simulink model "MPC3DoF_state_est"  (R2024b)
settings: Solver=VariableStepAuto  StartTime=0.0  StopTime=stop_time  RelTol=1e-3
model workspace (MAT data in the model file):
  com_error = 0
  controller_type : ControllerType (value not decoded)
  discrepancy = 0.5
  dtime = 0.3
  enable_turbulence = 0
  filter_update_time = 0.05
  g = 9.8
  inertia_error = 0
  lla_ref = [40.425869 -86.908066 187]
  mass_error = 0
  max_gimbal_rate = 5
  max_iter = 400
  max_throttle_rate = 0.5
  nominal_val = 5
  optimization_time = 0.3
  steps = 50
  stop_time = inf
  u0 = [0.443891402715 0]
  vehicle = Vehicle
  vehicle.m = 100000
  vehicle.L = 30
  vehicle.I = 30000000
  vehicle.Len = 60
  vehicle.max_gimbal = 0.174532925199
  vehicle.min_thrust = 440000
  vehicle.max_thrust = 2210000
  vehicle.Name = "Astra2"
  x0 = [100 100 0 0 1.57079632679 0]
  xf = [0 0 0 0 1.57079632679 0]
libraries: simulink_extras x4, aerolibanim x1, SignalEditorBlockLib x1
settings Model: Creator=alexa  LastModifiedBy=thatf

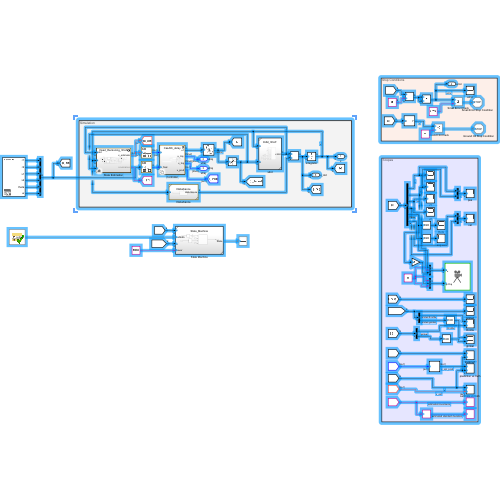
[thumbnail: Simulink's stored preview of the top-level diagram]
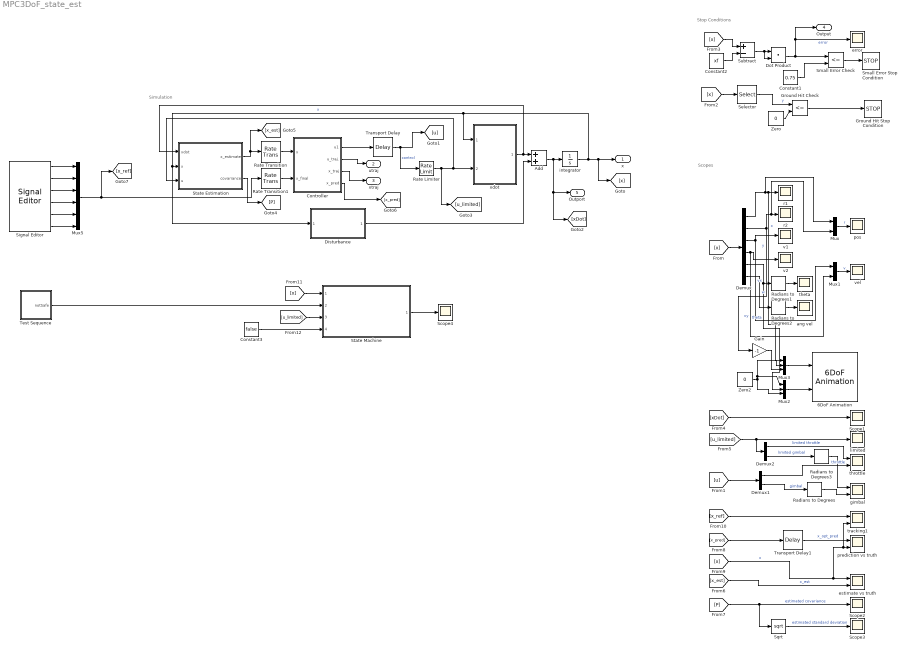
== system MPC3DoF_state_est ==
  note: Simulation
  note: Stop Conditions
  note: Scopes
  6DoF Animation : aerolibanim/6DoF Animation  u1=[-100 100 -100 100 -800 0]  u2=0.1  u3=10.0  u4=[0, 0, 0]  u5=Fixed position  u6=[0,80,-50]  u7=40  u8=on
  Add : Sum
  Constant1 : Constant  Value=0.75
  Constant2 : Constant  Value=xf
  Constant3 : Constant  Value=false
  Controller : Subsystem  Variant=on  VariantChoicesSpecifier={}  VariantChoicesEnumeration=ControllerType  VariantControlVariable=controller_type
  Demux : Demux  Outputs=6
  Demux1 : Demux  Outputs=2
  Demux2 : Demux  Outputs=2
  Disturbance : Subsystem  ReferencedSubsystem=Disturbance
  Dot Product : DotProduct  OutDataTypeStr=Inherit: Inherit via internal rule
  Gain : Gain  Gain=-1
  Ground Hit Check : RelationalOperator  Operator=<=  OutDataTypeStr=boolean  RndMeth=Simplest  InputSameDT=off
  Ground Hit Stop Condition : Stop
  Mux : Mux  Inputs=2
  Mux1 : Mux  Inputs=2
  Mux2 : Mux  Inputs=3
  Mux3 : Mux  Inputs=3
  Mux5 : Mux  Inputs=6
  Radians to Degrees{,1..3} (4 alike) : simulink_extras/Transformations/Radians to Degrees
  Rate Limiter : RateLimiter  RisingSlewLimit=[max_throttle_rate max_gimbal_rate]*100  FallingSlewLimit=[-max_throttle_rate -max_gimbal_rate]*100  SampleTimeMode=inherited  InitialCondition=u0
  Rate Transition : RateTransition  InitialCondition=x0  OutPortSampleTime=optimization_time
  Rate Transition1 : RateTransition  InitialCondition=xf  OutPortSampleTime=optimization_time
  Scope{1..4} (4 alike) : Scope
  Selector : Selector  InputPortWidth=6  IndexOptions=Index vector (dialog)  Indices=[2]  OutputSizes=1
  Signal Editor : SignalEditorBlockLib/Signal Editor  FileName=land_at_origin_scenario.mat  ActiveScenario=Scenario  ActiveSignal=w  IsBus=off  OutputBusObjectStr=Bus: BusObject  SampleTime=0  ZeroCross=off  OutputAfterFinalValue=Holding final value  Unit=inherit  PreserveSignalName=on  ApplySigPropsToAllScenarios=on  ApplySigPropsToAllSignals=on
  Small Error Check : RelationalOperator  Operator=<=  OutDataTypeStr=boolean  RndMeth=Simplest  InputSameDT=off
  Small Error Stop Condition : Stop
  Sqrt : Sqrt
  State Estimation : Subsystem  Variant=on  VariantChoicesSpecifier="[\"EKF_IMU_GPS_3DoF\", \"Perfect_State_Estimation\", \"Dead_Reckoning_3DoF\"]"  VariantControlMode=label  LabelModeActiveChoice=Dead_Reckoning_3DoF
  State Machine : Subsystem  ReferencedSubsystem=State_Machine
  Subtract : Sum  Inputs=+-
  Test Sequence : Test Sequence  TreatAsAtomicUnit=on
  Transport Delay : TransportDelay  DelayTime=optimization_time  InitialOutput=u0
  Transport Delay1 : TransportDelay  DelayTime=optimization_time  InitialOutput=x0'
  Zero : Constant  Value=0  OutDataTypeStr=Inherit: Inherit via back propagation
  Zero2 : Constant  Value=0  OutDataTypeStr=Inherit: Inherit via back propagation
  ang vel : Scope
  error : Scope
  estimate vs truth : Scope  NumInputPorts=2
  gimbal : Scope  NumInputPorts=2
  integrator : Integrator  InitialCondition=x0
  limited : Scope
  pos : Scope
  prediction vs truth : Scope  NumInputPorts=2
  r1 : Scope
  r2 : Scope
  theta : Scope
  throttle : Scope  NumInputPorts=2
  tracking1 : Scope  NumInputPorts=2
  v1 : Scope
  v2 : Scope
  vel : Scope
  xdot : Subsystem  ReferencedSubsystem=EoM_3DoF
  x : Outport  SignalName=x
  utraj : Outport  Port=2  SignalName=utraj
  xtraj : Outport  Port=3  SignalName=xtraj
  Output : Outport  Port=4  SignalName=error
  Outport : Outport  Port=5  SignalName=x_dot
  wires:
  xdot/1 -> State Estimation/1(xdot), Add/1
  integrator/1 -> xdot/1, State Estimation/2(x), Disturbance/1, x/1, [x]  "x"
  Controller/3(x_traj) -> xtraj/1
  Transport Delay/1 -> [u], Rate Limiter/1  "control"
  Mux/1 -> pos/1  "r"
  Demux/6 -> Radians to Degrees2/1  "w"
  Demux/3 -> v1/1, Mux1/1  "vx"
  Demux/2 -> Mux/2, r2/1, Gain/1  "y"
  Demux/5 -> Mux2/2, Radians to Degrees1/1  "theta"
  Demux/1 -> Mux/1, Mux3/1, r1/1  "x"
  Mux1/1 -> vel/1  "v"
  Demux/4 -> Mux1/2, v2/1  "vy"
  [x] -> Demux/1
  [u] -> Demux1/1
  Demux1/1 -> throttle/2  "throttle"
  Demux1/2 -> Radians to Degrees/1  "gimbal"
  Radians to Degrees/1 -> gimbal/2
  Radians to Degrees1/1 -> theta/1
  Radians to Degrees2/1 -> ang vel/1
  Controller/2(u_traj.) -> utraj/1
  Mux2/1 -> 6DoF Animation/2
  Mux3/1 -> 6DoF Animation/1
  Zero2/1 -> Mux2/1, Mux3/2, Mux2/3
  Gain/1 -> Mux3/3
  Add/1 -> integrator/1, [xDot], Outport/1
  Rate Transition/1 -> Controller/1(x)
  Disturbance/1 -> Add/2
  Controller/1(u1) -> Transport Delay/1
  Ground Hit Check/1 -> Ground Hit Stop Condition/1
  Constant1/1 -> Small Error Check/2
  Constant2/1 -> Subtract/2
  Selector/1 -> Ground Hit Check/1  "y"
  Dot Product/1 -> Output/1, error/1, Small Error Check/1  "error"
  Subtract/1 -> Dot Product/2, Dot Product/1
  [x] -> Selector/1
  Zero/1 -> Ground Hit Check/2
  [x] -> Subtract/1
  Small Error Check/1 -> Small Error Stop Condition/1
  [xDot] -> Scope1/1
  Rate Limiter/1 -> [u_limited], State Estimation/3(u), xdot/2
  [u_limited] -> Demux2/1, limited/1
  Rate Transition1/1 -> Controller/2(x_final)
  Demux2/1 -> throttle/1  "limited throttle"
  Demux2/2 -> Radians to Degrees3/1  "limited gimbal"
  Radians to Degrees3/1 -> gimbal/1
  Controller/4(x_pred) -> [x_pred]
  State Estimation/1(x_estimate) -> [x_est], Rate Transition/1
  State Estimation/2(covariance) -> [P]
  [x_est] -> estimate vs truth/2  "x_est"
  [P] -> Scope2/1, Sqrt/1  "estimated covariance"
  Sqrt/1 -> Scope3/1  "estimated standard deviation"
  Transport Delay1/1 -> prediction vs truth/1  "x_opt_pred"
  [x_pred] -> Transport Delay1/1
  [x] -> estimate vs truth/1, tracking1/2, prediction vs truth/2  "x"
  [x_ref] -> tracking1/1
  Mux5/1 -> Rate Transition1/1, [x_ref]
  Signal Editor/6 -> Mux5/6
  Signal Editor/1 -> Mux5/1
  Signal Editor/4 -> Mux5/4
  Signal Editor/5 -> Mux5/5
  Signal Editor/2 -> Mux5/2
  Signal Editor/3 -> Mux5/3
  [x] -> State Machine/1
  [u_limited] -> State Machine/3
  Test Sequence/1(notSafe) -> State Machine/2
  State Machine/1 -> Scope4/1
  Constant3/1 -> State Machine/4

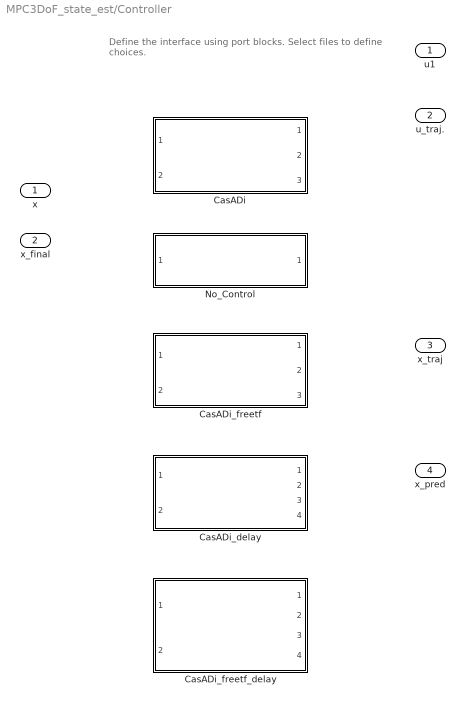
== system MPC3DoF_state_est/Controller ==
  note: Define the interface using port blocks.
      | Select files to define choices.
  x : Inport
  x_final : Inport  Port=2
  CasADi : Subsystem  VariantControl=controller_type == ControllerType.CasADi  ReferencedSubsystem=CasADi
  CasADi_delay : Subsystem  VariantControl=controller_type == ControllerType.CasADi_delay  ReferencedSubsystem=CasADi_delay
  CasADi_freetf : Subsystem  VariantControl=controller_type == ControllerType.CasADi_freetf  ReferencedSubsystem=CasADi_freetf
  CasADi_freetf_delay : Subsystem  VariantControl=controller_type == ControllerType.CasADi_freetf_delay  ReferencedSubsystem=CasADi_freetf_delay
  No_Control : Subsystem  VariantControl=controller_type == ControllerType.No_Control  ReferencedSubsystem=No_Control
  u1 : Outport
  u_traj. : Outport  Port=2
  x_traj : Outport  Port=3
  x_pred : Outport  Port=4

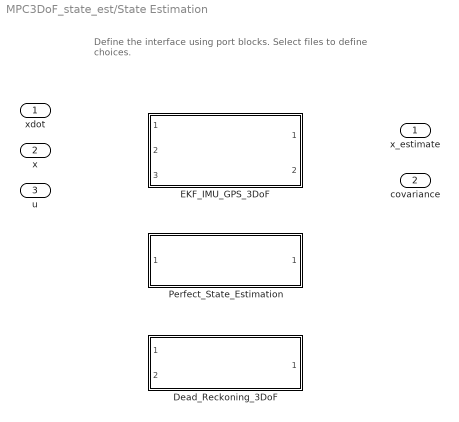
== system MPC3DoF_state_est/State Estimation ==
  note: Define the interface using port blocks.
      | Select files to define choices.
  xdot : Inport
  x : Inport  Port=2
  u : Inport  Port=3
  Dead_Reckoning_3DoF : Subsystem  VariantControl=Dead_Reckoning_3DoF  ReferencedSubsystem=Dead_Reckoning_3DoF
  EKF_IMU_GPS_3DoF : Subsystem  VariantControl=EKF_IMU_GPS_3DoF  ReferencedSubsystem=EKF_IMU_GPS_3DoF
  Perfect_State_Estimation : Subsystem  VariantControl=Perfect_State_Estimation  ReferencedSubsystem=Perfect_State_Estimation
  x_estimate : Outport
  covariance : Outport  Port=2

== stateflow chart MPC3DoF_state_est/Test Sequence ==
  state Scenario_1
    state step_1
    state step_2
      notSafe = true;
    (default) -> step_1
    step_1 -> step_2 : [
        | after(5, sec)
        | ]
  (default) -> Scenario_1 : {assert(Active_Scenario_Index == 1,'The value of Scenario Parameter ''Active_Scenario_Index'' is not valid. Use the index of the scenario to specify it.')}
  data: Active_Scenario_Index parameter =1; notSafe output
